simulink model "DCmotor"  (R2016a)
settings: Solver=ode23t  StartTime=0.0  StopTime=10.0  RelTol=1e-3  AbsTol=1e-3
libraries: fl_lib x12, nesl_utility x3
settings Model: Creator=STF2972  LastModifiedBy=STF2972
settings GRTTargetCC: GeneratePreprocessorConditionals=Use local settings
settings SimscapeCC: SimscapeLogType=all  SimscapeLogDataHistory=10000

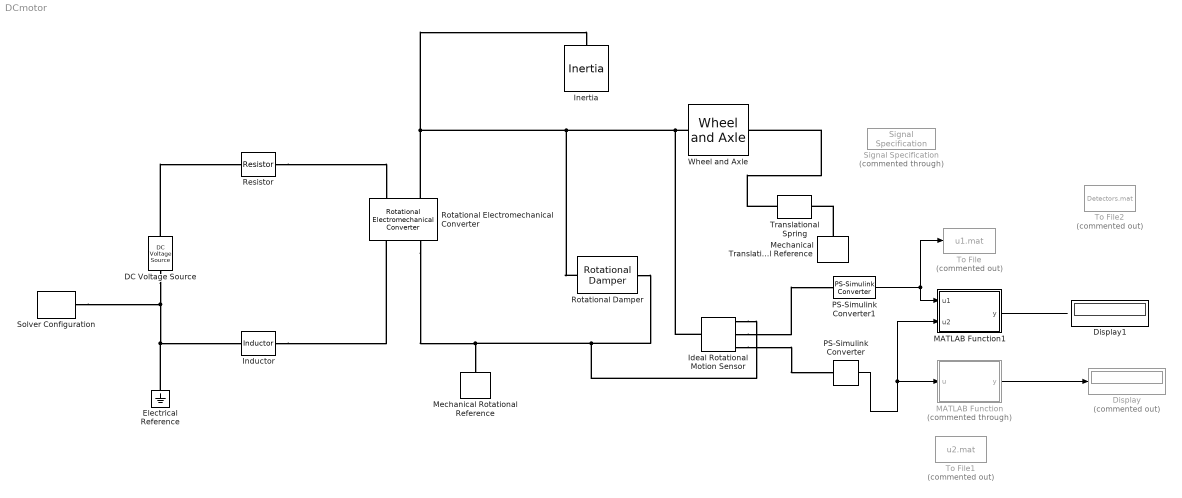
== system DCmotor ==
  DC Voltage Source : fl_lib/Electrical/Electrical Sources/DC Voltage Source  v0=5 V
  Display : Display  Commented=on
  Display1 : Display
  Electrical Reference : fl_lib/Electrical/Electrical Elements/Electrical Reference
  Ideal Rotational Motion Sensor : fl_lib/Mechanical/Mechanical Sensors/Ideal Rotational Motion Sensor  offset=0 rad
  Inductor : fl_lib/Electrical/Electrical Elements/Inductor  l=1e-6 H  r=0 Ohm  g=1e-9 1/Ohm  i_specify=off  i_priority=None  i=0 A  v_specify=off  v_priority=None  v=0 V  i_L_specify=off  i_L_priority=High  i_L=0 A
  Inertia : fl_lib/Mechanical/Rotational Elements/Inertia  inertia=0.01 kg*m^2  w_specify=off  w_priority=High  w=0 rad/s  t_specify=off  t_priority=None  t=0 N*m
  MATLAB Function : MATLAB Function  Commented=through  TreatAsAtomicUnit=on
  MATLAB Function1 : MATLAB Function  TreatAsAtomicUnit=on
  Mechanical Rotational Reference : fl_lib/Mechanical/Rotational Elements/Mechanical Rotational Reference
  Mechanical Translational Reference : fl_lib/Mechanical/Translational Elements/Mechanical Translational Reference
  PS-Simulink Converter : nesl_utility/PS-Simulink Converter  PhysicalDomain=network_engine_domain  SubClassName=ps_output  LeftPortType=input  RightPortType=output  PseudoPeriodic=off  Frequencies=[]  Unit=deg  AffineConversion=off
  PS-Simulink Converter1 : nesl_utility/PS-Simulink Converter  PhysicalDomain=network_engine_domain  SubClassName=ps_output  LeftPortType=input  RightPortType=output  PseudoPeriodic=off  Frequencies=[]  Unit=1  AffineConversion=off
  Resistor : fl_lib/Electrical/Electrical Elements/Resistor  R=1 Ohm  i_specify=off  i_priority=None  i=0 A  v_specify=off  v_priority=None  v=0 V
  Rotational Electromechanical Converter : fl_lib/Electrical/Electrical Elements/Rotational Electromechanical Converter  K=0.1 V/(rad/s)  i_specify=off  i_priority=None  i=0 A  v_specify=off  v_priority=None  v=0 V  t_specify=off  t_priority=None  t=0 N*m  w_specify=off  w_priority=None  w=0 rad/s
  Rotational Damper : fl_lib/Mechanical/Rotational Elements/Rotational Damper  D=0.001 N*m/(rad/s)  w_specify=off  w_priority=None  w=0 rad/s  t_specify=off  t_priority=None  t=0 N*m
  Signal Specification : SignalSpecification  Commented=through
  Solver Configuration : nesl_utility/Solver Configuration  PhysicalDomain=network_engine_domain  SubClassName=solver  LeftPortType=input  RightPortType=generic  Accelerate=off  Tones=[]  Harmonics=[]  SimulateNoise=off  Profile=off  UseLocalSampling=off  EnableSwitchedLinearOptims=on  FrequencyDomain=off  UseCCode=off  RelTol=0.001  AbsTol=1e-06  MinStep=1e-09  ToWorkspace=off  RevertToSquareIcSolve=off  NumHomotopyIterations=100  PhasorMode=off  PhasorModeNumHarmonics=1  OverrideAbsTol=off  DoDC=off  ResidualTolerance=1e-09  UseLocalSolver=off  LocalSolverChoice=NE_BACKWARD_EULER_ADVANCER  LocalSolverSampleTime=0.001  DoFixedCost=off  MaxNonlinIter=3  MaxModeIter=2  LinearAlgebra=Sparse  DelaysMemoryBudget=1024  AutomaticFiltering=on  FilteringTimeConstant=0.001
  To File : ToFile  Commented=on  Filename=u1.mat  MatrixName=u_1
  To File1 : ToFile  Commented=on  Filename=u2.mat  MatrixName=u_2
  To File2 : ToFile  Commented=on  Filename=Detectors.mat  MatrixName=detectorSet
  Translational Spring : fl_lib/Mechanical/Translational Elements/Translational Spring  spr_rate=1000 N/m  v_specify=off  v_priority=None  v=0 m/s  f_specify=off  f_priority=None  f=0 N  x_specify=off  x_priority=High  x=0 m
  Wheel and Axle : fl_lib/Mechanical/Mechanisms/Wheel and Axle  R=0.05 m  or=1  t_specify=off  t_priority=None  t=0 N*m  f_specify=off  f_priority=None  f=0 N
  wires:
  PS-Simulink Converter/1 -> MATLAB Function/1(u), MATLAB Function1/2(u2)
  PS-Simulink Converter1/1 -> MATLAB Function1/1(u1), To File/1
  MATLAB Function/1(y) -> Display/1
  ? -> Display1/1
  MATLAB Function1/1(y) -> ?
  connections:
  DC Voltage Source/LConn1 -- Resistor/LConn1
  Resistor/RConn1 -- Rotational Electromechanical Converter/LConn1
  DC Voltage Source/RConn1 -- Solver Configuration/RConn1 -- Electrical Reference/LConn1 -- Inductor/LConn1
  Inductor/RConn1 -- Rotational Electromechanical Converter/RConn1
  Rotational Electromechanical Converter/RConn2 -- Ideal Rotational Motion Sensor/RConn1 -- Rotational Damper/RConn1 -- Mechanical Rotational Reference/LConn1
  Rotational Electromechanical Converter/LConn2 -- Ideal Rotational Motion Sensor/LConn1 -- Wheel and Axle/LConn1 -- Rotational Damper/LConn1 -- Inertia/LConn1
  Translational Spring/LConn1 -- Wheel and Axle/RConn1
  Mechanical Translational Reference/LConn1 -- Translational Spring/RConn1
  Ideal Rotational Motion Sensor/RConn3 -- PS-Simulink Converter/LConn1
  Ideal Rotational Motion Sensor/RConn2 -- PS-Simulink Converter1/LConn1

== matlab function DCmotor/MATLAB Function1 ==
  data: u1 input; u2 input; y output [0..50]

function y = fcn(u1,u2)

%% #codegen
coder.extrinsic('clc');
persistent detSet;
if isempty(detSet)
detSet=zeros(1,3);
end
coder.varsize('detSet',[30000000 3]);

x_1=11.4591559045;
x_2 =11.45915590;


y_1=4e-10; 
y_2=-4e-10; 
%%Distance measures
dist_min=0;
temp_dist=0;
rDet=0;
c_s1 =(x_1+x_2)/2;
c_s2=(y_1+y_2)/2;

if (abs(y_1-y_2)>abs(x_1-x_2))
    rs =abs(x_1-x_2);
else 
    rs =abs(y_1-y_2);
end 
% center of self and the radious 
circle(c_s1, c_s2,abs(y_1-y_2));
%drawCircle(c_s1, c_s2,rs);
%filledCircle([c_s1,c_s2],rs,1000,'r')
%Until N ==m_max
N=0; % count of not self
 %# of detectors


p=0.5; % default probability 
x=0; % %Selected point /occarance 
n=0; % sample size/ total number of data
m =0; % detected occurances
n_sample=10; % predefined sample size



% Detector set map(Key value pair diameter)
%detSet = containers.Map('KeyType','double','ValueType','double');
% coder.extrinsic(detset);
% detSet = java.util.Hashtable;
% bool =exist(detSet);
% if bool
%detSet = zeros(1,3);
%detSet= [1 1 1];
%detSet=[detSet; o];
% end 
% Estimated coverage 99% 
%%%% Hyppthesis testing %%%%
m_max =max(5/p, 5/(1-p));
z_alpha =3.49;
% Sample a point 
i=0;


% %%
% %two dimensional space 
 
 a=u1;
 b =u2;
 
%  d=abs(sqrt(((a-c_s2).^2+(b-c_s1).^2))-rs);
%   e= [a d b];
% 
%   detSet=[detSet; e]
%   y=detSet
% 
%  if(abs (sqrt(((b-c_s2)^2+(a-c_s1)^2))-rs))>rs % Euclidean distance 
%         %%--------not-self-------
%         %%                                                                                                      
%         N=N+1; % count not self sample
%      
%             % addthe first detector to the map
%             c=abs(sqrt(((b-c_s2)^2+(a-c_s1)^2))-rs);
%             b= [a b c];
%             detSet=[detSet; b];
%             [rows cols] =size(detSet);
%  end 

 if(a>0.1 && b>0.1)      
if (N<m_max) % exit criterion 
   n =n+1; % count the sample size
   if(abs (sqrt(((b-c_s2)^2+(a-c_s1)^2))-rs))>rs % Euclidean distance 
        %%--------not-self-------
        %%                                                                                                      
        N=N+1; % count not self sample
         
        if size(detSet,1)==1 % first detector    
            % addthe first detector to the map
            c=sqrt(((b-c_s2)^2+(a-c_s1)^2))-rs;
            detSet=[detSet; [a b c]];
            %y=detSet;
            %xlswrite('detectors.xlsx',detSet);
           
            circle(a,b,c);
           
 
       
            
        else
        %find the closest detector
           rDet=0;
           
            %finding the minimum distance to the point selected
            for j=1: size(detSet,1)              
                temp_dist = (b-detSet(j,2))^2+(a-detSet(j,1))^2;
                if(j>1)
                    if(temp_dist<dist_min)
                    dist_min=temp_dist;
                    rDet =detSet(j,3);
                    end
                else 
                    dist_min =temp_dist;
                    rDet =detSet(j,3);
                end 
                
            end 
                %% check if it is out side of the closest detector
                     
                   
            
            %Check if it is within the raduis of the closest detector
            
        
            %% Covered? yes 
        
            if rDet>dist_min
                 %% Covered? yes
                m=m+1; % count covered sample
                p =N/n; % probability of not self
                q= 1-N/n;
                z=m/sqrt(n*p*q)-sqrt(n*p/q); % evaluate z score
                if z<z_alpha % not enough coverage
                    if(N==n_sample) 
                        %% Accept all saved candidates as new detectors
                        N=0;
                        m=0;
                    
                        
                    end 
                else %enough coverage
                    N=m_max+1; % exist the function
                end 
            else 
                %% Covered? No : save the candidate
                detSet=[detSet; [a b sqrt(dist_min)]];
               
                circle(a,b,sqrt(dist_min));
               
            end    
        end 
    end 
       
end 
 end 
y =a;
%This assignment writes a 'double' value into a 'embedded.fi {int16}' type. Code generation does not support changing types through assignment. Check preceding assignments or input type specifications for type mismatches.


% 
 

 function circle(x,y,r)
%x and y are the coordinates of the center of the circle
%r is the radius of the circle
%0.01 is the angle step, bigger values will draw the circle faster but
%you might notice imperfections (not very smooth)
ang=0:0.01:2*pi; 
xp=r*cos(ang);
yp=r*sin(ang);
plot(x+xp,y+yp);
hold on
function h = filledCircle(center,r,N,color)
%---------------------------------------------------------------------------------------------
% FILLEDCIRCLE Filled circle drawing
% 
% filledCircle(CENTER,R,N,COLOR) draws a circle filled with COLOR that 
% has CENTER as its center and R as its radius, by using N points on the 
% periphery.
%
% Usage Examples,
%
% filledCircle([1,3],3,1000,'b'); 
% filledCircle([2,4],2,1000,'r');
%
% Sadik Hava <sadik.hava@gmail.com>
% May, 2010
%
% Inspired by: circle.m [Author: Zhenhai Wang]
%---------------------------------------------------------------------------------------------

THETA=linspace(0,2*pi,N);
RHO=ones(1,N)*r;
[X,Y] = pol2cart(THETA,RHO);
X=X+center(1);
Y=Y+center(2);
h=fill(X,Y,color);
axis square;


% COPYRIGHT STUFF... :D (Since I am modifying Zhenhai's code.)
%
% Copyright (c) 2002, Zhenhai Wang
% All rights reserved.
% 
% Redistribution and use in source and binary forms, with or without 
% modification, are permitted provided that the following conditions are 
% met:
% 
%     * Redistributions of source code must retain the above copyright 
%       notice, this list of conditions and the following disclaimer.
%     * Redistributions in binary form must reproduce the above copyright 
%       notice, this list of conditions and the following disclaimer in 
%       the documentation and/or other materials provided with the distribution
%       
% THIS SOFTWARE IS PROVIDED BY THE COPYRIGHT HOLDERS AND CONTRIBUTORS "AS IS" 
% AND ANY EXPRESS OR IMPLIED WARRANTIES, INCLUDING, BUT NOT LIMITED TO, THE 
% IMPLIED WARRANTIES OF MERCHANTABILITY AND FITNESS FOR A PARTICULAR PURPOSE 
% ARE DISCLAIMED. IN NO EVENT SHALL THE COPYRIGHT OWNER OR CONTRIBUTORS BE 
% LIABLE FOR ANY DIRECT, INDIRECT, INCIDENTAL, SPECIAL, EXEMPLARY, OR 
% CONSEQUENTIAL DAMAGES (INCLUDING, BUT NOT LIMITED TO, PROCUREMENT OF 
% SUBSTITUTE GOODS OR SERVICES; LOSS OF USE, DATA, OR PROFITS; OR BUSINESS 
% INTERRUPTION) HOWEVER CAUSED AND ON ANY THEORY OF LIABILITY, WHETHER IN 
% CONTRACT, STRICT LIABILITY, OR TORT (INCLUDING NEGLIGENCE OR OTHERWISE) 
% ARISING IN ANY WAY OUT OF THE USE OF THIS SOFTWARE, EVEN IF ADVISED OF THE 
% POSSIBILITY OF SUCH DAMAGE.

== matlab function DCmotor/MATLAB Function ==
  data: u input; y output [1..2]
function y = fcn(u)
%#codegen
coder.extrinsic('clc');
persistent d n;
if isempty(n)
n=0;
end
% size(d,1)
assert(n<=10000);
coder.varsize('d',[30000000 3]);
b=[u u+1 u+2];
if isempty(d)
    n=1;
d=zeros(n,3);
else 
    n =size(d,1);
    d=[b;d]

end

y = u;
